simulink subsystem "target_motion_subsystem"  (R2021b)
settings: Solver=VariableStepAuto  StartTime=0.0  StopTime=10.0  RelTol=1e-3
values from neighbouring files (symbols this model uses):
  l_T0 = -2.5*d2r    (= -0.0436332312999)    [PN_Guidance_matlab.m]
  V_T = 600    [PN_Guidance_matlab.m]
  X_M0 = 2000    [PN_Guidance_matlab.m]
  X_T0 = 100    [PN_Guidance_matlab.m]
  Z_T0 = 20000    [PN_Guidance_matlab.m]
settings Model: Creator=rocke  LastModifiedBy=rocke

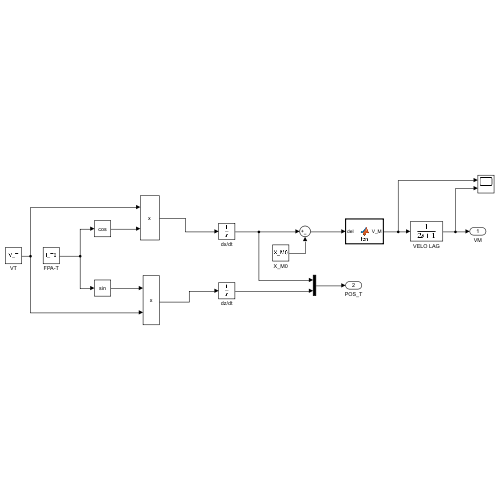
[thumbnail: Simulink's stored preview of the top-level diagram]
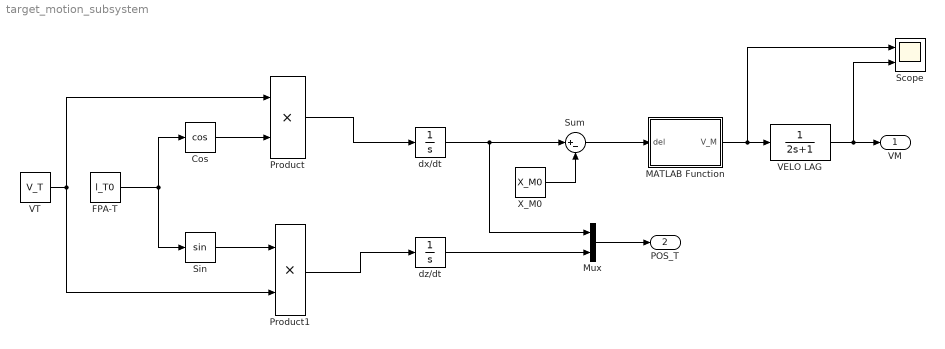
== system target_motion_subsystem ==
  Cos : Trigonometry  Operator=cos
  FPA-T : Constant  Value=l_T0
  MATLAB Function : MATLAB Function  TreatAsAtomicUnit=on
  Mux : Mux  Inputs=2
  Product : Product
  Product1 : Product
  Scope : Scope  NumInputPorts=2
  Sin : Trigonometry
  Sum : Sum  Inputs=|+-
  VELO LAG : TransferFcn  Denominator=[2 1]
  VT : Constant  Value=V_T
  X_M0 : Constant  Value=X_M0
  dx/dt : Integrator  InitialCondition=X_T0
  dz/dt : Integrator  InitialCondition=Z_T0
  VM : Outport
  POS_T : Outport  Port=2
  wires:
  Sin/1 -> Product1/1
  Cos/1 -> Product/2
  Product1/1 -> dz/dt/1
  Product/1 -> dx/dt/1
  X_M0/1 -> Sum/2
  Mux/1 -> POS_T/1
  Sum/1 -> MATLAB Function/1(del)
  VELO LAG/1 -> Scope/2, VM/1
  FPA-T/1 -> Sin/1, Cos/1
  MATLAB Function/1(V_M) -> Scope/1, VELO LAG/1
  dz/dt/1 -> Mux/2
  VT/1 -> Product/1, Product1/2
  dx/dt/1 -> Mux/1, Sum/1

== matlab function target_motion_subsystem/MATLAB Function ==
  data: del input; V_M output
function V_M = fcn(del)
%#codegen

persistent f 
persistent Vel

if isempty(f)
    f=0;
end
if isempty(Vel)
    Vel=0;
end

if f==0 && del > -200
    f=1;
    Vel=1021;
end

V_M=Vel;
